simulink model "PhysicalEverSimmer"  (R2026a)
settings: Solver=VariableStepAuto  StopTime=14400
undefined symbols (not defined in the file or in its folder): ES_PackRate_bph, ES_PrepRate_bph, ES_QCRate_bph, ES_Resupply_bph, Fault_T_Cell1, Fault_T_Cell2, Fault_T_Cell3, Recipe_Block_s, Recipe_Count, Resupply_Cutoff_T, Transport_Latency_s, Transport_Rate_bph
(part 1 of 2)
settings Model: DataDictionary=PhysicalEverSimmerData.sldd  Creator=sarah  LastModifiedBy=sarah

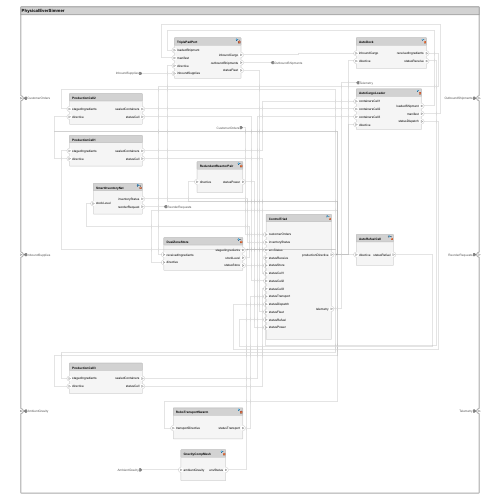
[thumbnail: Simulink's stored preview of the top-level diagram]
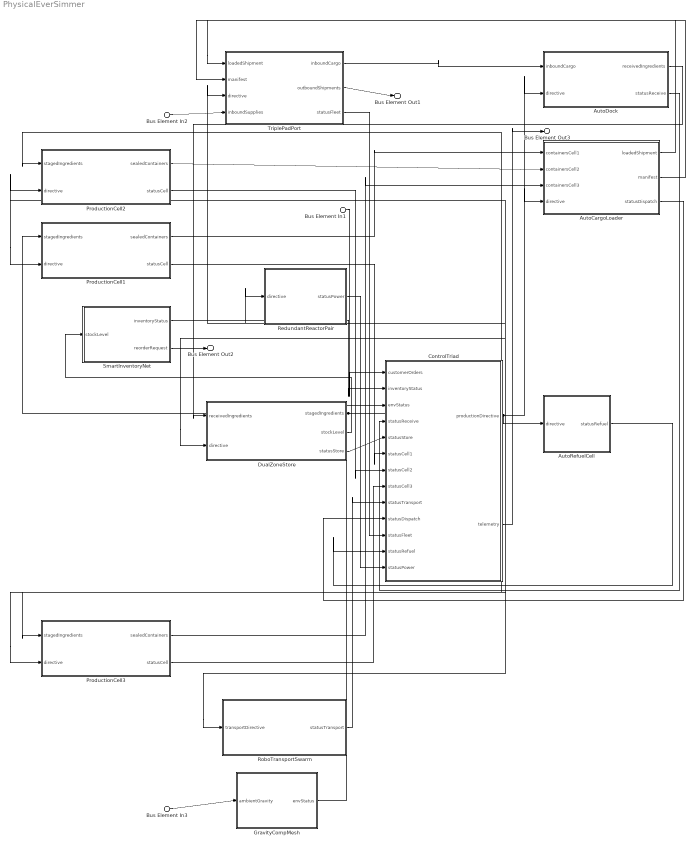
== system PhysicalEverSimmer ==
  Bus Element In1 : Inport  PortName=CustomerOrders
  Bus Element In2 : Inport  Port=2  PortName=InboundSupplies
  Bus Element In3 : Inport  Port=3  PortName=AmbientGravity
  AutoCargoLoader : Subsystem
      settings: PortSchema="{\"entries\":[{\"content\":{\"headerSize\":26,\"margin\":15,\"minimumSpacing\":25,\"sides\":[{\"content\":{\"connectorIds\":[\"In1\",\"In2\",\"In3\",\"In4\"]},\"type\":\"ConnectorPlacement.EquallySpacedRectSide\",\"uuid\":\"f830f98a-8e8b-4468-adf4-d6eab644987f\"},{\"content\":{\"connectorIds\":[\"Out1\",\"Out2\",\"Out3\"],\"side\":\"RIGHT\"},\"type\":\"ConnectorPlacement.EquallySpacedRectSide\",\"uuid\":\"7e0d0116-b3ba-4668-b638-30d0f54ba087\"},{\"content\":{\"side\":\"TOP\"},\"type\":\"ConnectorPlacement.EquallySpacedRectSide\",\"uuid\":\"7b4146d3-46d2-45ca-8c34-b106f0d8cedd\"}]},\"type\":\"ConnectorPlacement.EquallySpacedConnector\",\"uuid\":\"3d911b2d-a78f-42ea-b869-5e09982d9f54\"}],\"packageUris\":[\"http://schema.mathworks.com/mf0/Connector/R2020b\"],\"version\":\"1.0\"}"
  AutoDock : Subsystem
      settings: PortSchema="{\"entries\":[{\"content\":{\"headerSize\":26,\"margin\":15,\"minimumSpacing\":25,\"sides\":[{\"content\":{\"connectorIds\":[\"In1\",\"In2\"]},\"type\":\"ConnectorPlacement.EquallySpacedRectSide\",\"uuid\":\"f830f98a-8e8b-4468-adf4-d6eab644987f\"},{\"content\":{\"connectorIds\":[\"Out1\",\"Out2\"],\"side\":\"RIGHT\"},\"type\":\"ConnectorPlacement.EquallySpacedRectSide\",\"uuid\":\"7e0d0116-b3ba-4668-b638-30d0f54ba087\"},{\"content\":{\"side\":\"TOP\"},\"type\":\"ConnectorPlacement.EquallySpacedRectSide\",\"uuid\":\"7b4146d3-46d2-45ca-8c34-b106f0d8cedd\"}]},\"type\":\"ConnectorPlacement.EquallySpacedConnector\",\"uuid\":\"3d911b2d-a78f-42ea-b869-5e09982d9f54\"}],\"packageUris\":[\"http://schema.mathworks.com/mf0/Connector/R2020b\"],\"version\":\"1.0\"}"
  AutoRefuelCell : Subsystem
      settings: PortSchema="{\"entries\":[{\"content\":{\"headerSize\":26,\"margin\":15,\"minimumSpacing\":25,\"sides\":[{\"content\":{\"connectorIds\":[\"In1\"]},\"type\":\"ConnectorPlacement.EquallySpacedRectSide\",\"uuid\":\"f830f98a-8e8b-4468-adf4-d6eab644987f\"},{\"content\":{\"connectorIds\":[\"Out1\"],\"side\":\"RIGHT\"},\"type\":\"ConnectorPlacement.EquallySpacedRectSide\",\"uuid\":\"7e0d0116-b3ba-4668-b638-30d0f54ba087\"},{\"content\":{\"side\":\"TOP\"},\"type\":\"ConnectorPlacement.EquallySpacedRectSide\",\"uuid\":\"7b4146d3-46d2-45ca-8c34-b106f0d8cedd\"}]},\"type\":\"ConnectorPlacement.EquallySpacedConnector\",\"uuid\":\"3d911b2d-a78f-42ea-b869-5e09982d9f54\"}],\"packageUris\":[\"http://schema.mathworks.com/mf0/Connector/R2020b\"],\"version\":\"1.0\"}"
  ControlTriad : Subsystem
      settings: PortSchema="{\"entries\":[{\"content\":{\"headerSize\":26,\"margin\":15,\"minimumSpacing\":25,\"sides\":[{\"content\":{\"connectorIds\":[\"In1\",\"In2\",\"In3\",\"In4\",\"In5\",\"In6\",\"In7\",\"In8\",\"In9\",\"In10\",\"In11\",\"In12\",\"In13\"]},\"type\":\"ConnectorPlacement.EquallySpacedRectSide\",\"uuid\":\"f830f98a-8e8b-4468-adf4-d6eab644987f\"},{\"content\":{\"connectorIds\":[\"Out1\",\"Out2\"],\"side\":\"RIGHT\"},\"type\":\"ConnectorPlacement.EquallySpacedRectSide\",\"uuid\":\"7e0d0116-b3ba-4668-b638-30d0f54ba087\"},{\"content\":{\"side\":\"TOP\"},\"type\":\"ConnectorPlacement.EquallySpacedRectSide\",\"uuid\":\"7b4146d3-46d2-45ca-8c34-b106f0d8cedd\"}]},\"type\":\"ConnectorPlacement.EquallySpacedConnector\",\"uuid\":\"3d911b2d-a78f-42ea-b869-5e09982d9f54\"}],\"packageUris\":[\"http://schema.mathworks.com/mf0/Connector/R2020b\"],\"version\":\"1.0\"}"
  DualZoneStore : Subsystem
      settings: PortSchema="{\"entries\":[{\"content\":{\"headerSize\":26,\"margin\":15,\"minimumSpacing\":25,\"sides\":[{\"content\":{\"connectorIds\":[\"In1\",\"In2\"]},\"type\":\"ConnectorPlacement.EquallySpacedRectSide\",\"uuid\":\"f830f98a-8e8b-4468-adf4-d6eab644987f\"},{\"content\":{\"connectorIds\":[\"Out1\",\"Out2\",\"Out3\"],\"side\":\"RIGHT\"},\"type\":\"ConnectorPlacement.EquallySpacedRectSide\",\"uuid\":\"7e0d0116-b3ba-4668-b638-30d0f54ba087\"},{\"content\":{\"side\":\"TOP\"},\"type\":\"ConnectorPlacement.EquallySpacedRectSide\",\"uuid\":\"7b4146d3-46d2-45ca-8c34-b106f0d8cedd\"}]},\"type\":\"ConnectorPlacement.EquallySpacedConnector\",\"uuid\":\"3d911b2d-a78f-42ea-b869-5e09982d9f54\"}],\"packageUris\":[\"http://schema.mathworks.com/mf0/Connector/R2020b\"],\"version\":\"1.0\"}"
  GravityCompMesh : Subsystem
      settings: PortSchema="{\"entries\":[{\"content\":{\"headerSize\":26,\"margin\":15,\"minimumSpacing\":25,\"sides\":[{\"content\":{\"connectorIds\":[\"In1\"]},\"type\":\"ConnectorPlacement.EquallySpacedRectSide\",\"uuid\":\"f830f98a-8e8b-4468-adf4-d6eab644987f\"},{\"content\":{\"connectorIds\":[\"Out1\"],\"side\":\"RIGHT\"},\"type\":\"ConnectorPlacement.EquallySpacedRectSide\",\"uuid\":\"7e0d0116-b3ba-4668-b638-30d0f54ba087\"},{\"content\":{\"side\":\"TOP\"},\"type\":\"ConnectorPlacement.EquallySpacedRectSide\",\"uuid\":\"7b4146d3-46d2-45ca-8c34-b106f0d8cedd\"}]},\"type\":\"ConnectorPlacement.EquallySpacedConnector\",\"uuid\":\"3d911b2d-a78f-42ea-b869-5e09982d9f54\"}],\"packageUris\":[\"http://schema.mathworks.com/mf0/Connector/R2020b\"],\"version\":\"1.0\"}"
  ProductionCell1 : Subsystem
      settings: PortSchema="{\"entries\":[{\"content\":{\"headerSize\":26,\"margin\":15,\"minimumSpacing\":25,\"sides\":[{\"content\":{\"connectorIds\":[\"In1\",\"In2\"]},\"type\":\"ConnectorPlacement.EquallySpacedRectSide\",\"uuid\":\"f830f98a-8e8b-4468-adf4-d6eab644987f\"},{\"content\":{\"connectorIds\":[\"Out1\",\"Out2\"],\"side\":\"RIGHT\"},\"type\":\"ConnectorPlacement.EquallySpacedRectSide\",\"uuid\":\"7e0d0116-b3ba-4668-b638-30d0f54ba087\"},{\"content\":{\"side\":\"TOP\"},\"type\":\"ConnectorPlacement.EquallySpacedRectSide\",\"uuid\":\"7b4146d3-46d2-45ca-8c34-b106f0d8cedd\"}]},\"type\":\"ConnectorPlacement.EquallySpacedConnector\",\"uuid\":\"3d911b2d-a78f-42ea-b869-5e09982d9f54\"}],\"packageUris\":[\"http://schema.mathworks.com/mf0/Connector/R2020b\"],\"version\":\"1.0\"}"
  ProductionCell2 : Subsystem
      settings: PortSchema="{\"entries\":[{\"content\":{\"headerSize\":26,\"margin\":15,\"minimumSpacing\":25,\"sides\":[{\"content\":{\"connectorIds\":[\"In1\",\"In2\"]},\"type\":\"ConnectorPlacement.EquallySpacedRectSide\",\"uuid\":\"f830f98a-8e8b-4468-adf4-d6eab644987f\"},{\"content\":{\"connectorIds\":[\"Out1\",\"Out2\"],\"side\":\"RIGHT\"},\"type\":\"ConnectorPlacement.EquallySpacedRectSide\",\"uuid\":\"7e0d0116-b3ba-4668-b638-30d0f54ba087\"},{\"content\":{\"side\":\"TOP\"},\"type\":\"ConnectorPlacement.EquallySpacedRectSide\",\"uuid\":\"7b4146d3-46d2-45ca-8c34-b106f0d8cedd\"}]},\"type\":\"ConnectorPlacement.EquallySpacedConnector\",\"uuid\":\"3d911b2d-a78f-42ea-b869-5e09982d9f54\"}],\"packageUris\":[\"http://schema.mathworks.com/mf0/Connector/R2020b\"],\"version\":\"1.0\"}"
  ProductionCell3 : Subsystem
      settings: PortSchema="{\"entries\":[{\"content\":{\"headerSize\":26,\"margin\":15,\"minimumSpacing\":25,\"sides\":[{\"content\":{\"connectorIds\":[\"In1\",\"In2\"]},\"type\":\"ConnectorPlacement.EquallySpacedRectSide\",\"uuid\":\"f830f98a-8e8b-4468-adf4-d6eab644987f\"},{\"content\":{\"connectorIds\":[\"Out1\",\"Out2\"],\"side\":\"RIGHT\"},\"type\":\"ConnectorPlacement.EquallySpacedRectSide\",\"uuid\":\"7e0d0116-b3ba-4668-b638-30d0f54ba087\"},{\"content\":{\"side\":\"TOP\"},\"type\":\"ConnectorPlacement.EquallySpacedRectSide\",\"uuid\":\"7b4146d3-46d2-45ca-8c34-b106f0d8cedd\"}]},\"type\":\"ConnectorPlacement.EquallySpacedConnector\",\"uuid\":\"3d911b2d-a78f-42ea-b869-5e09982d9f54\"}],\"packageUris\":[\"http://schema.mathworks.com/mf0/Connector/R2020b\"],\"version\":\"1.0\"}"
  RedundantReactorPair : Subsystem
      settings: PortSchema="{\"entries\":[{\"content\":{\"headerSize\":26,\"margin\":15,\"minimumSpacing\":25,\"sides\":[{\"content\":{\"connectorIds\":[\"In1\"]},\"type\":\"ConnectorPlacement.EquallySpacedRectSide\",\"uuid\":\"f830f98a-8e8b-4468-adf4-d6eab644987f\"},{\"content\":{\"connectorIds\":[\"Out1\"],\"side\":\"RIGHT\"},\"type\":\"ConnectorPlacement.EquallySpacedRectSide\",\"uuid\":\"7e0d0116-b3ba-4668-b638-30d0f54ba087\"},{\"content\":{\"side\":\"TOP\"},\"type\":\"ConnectorPlacement.EquallySpacedRectSide\",\"uuid\":\"7b4146d3-46d2-45ca-8c34-b106f0d8cedd\"}]},\"type\":\"ConnectorPlacement.EquallySpacedConnector\",\"uuid\":\"3d911b2d-a78f-42ea-b869-5e09982d9f54\"}],\"packageUris\":[\"http://schema.mathworks.com/mf0/Connector/R2020b\"],\"version\":\"1.0\"}"
  RoboTransportSwarm : Subsystem
      settings: PortSchema="{\"entries\":[{\"content\":{\"headerSize\":26,\"margin\":15,\"minimumSpacing\":25,\"sides\":[{\"content\":{\"connectorIds\":[\"In1\"]},\"type\":\"ConnectorPlacement.EquallySpacedRectSide\",\"uuid\":\"f830f98a-8e8b-4468-adf4-d6eab644987f\"},{\"content\":{\"connectorIds\":[\"Out1\"],\"side\":\"RIGHT\"},\"type\":\"ConnectorPlacement.EquallySpacedRectSide\",\"uuid\":\"7e0d0116-b3ba-4668-b638-30d0f54ba087\"},{\"content\":{\"side\":\"TOP\"},\"type\":\"ConnectorPlacement.EquallySpacedRectSide\",\"uuid\":\"7b4146d3-46d2-45ca-8c34-b106f0d8cedd\"}]},\"type\":\"ConnectorPlacement.EquallySpacedConnector\",\"uuid\":\"3d911b2d-a78f-42ea-b869-5e09982d9f54\"}],\"packageUris\":[\"http://schema.mathworks.com/mf0/Connector/R2020b\"],\"version\":\"1.0\"}"
  SmartInventoryNet : Subsystem
      settings: PortSchema="{\"entries\":[{\"content\":{\"headerSize\":26,\"margin\":15,\"minimumSpacing\":25,\"sides\":[{\"content\":{\"connectorIds\":[\"In1\"]},\"type\":\"ConnectorPlacement.EquallySpacedRectSide\",\"uuid\":\"f830f98a-8e8b-4468-adf4-d6eab644987f\"},{\"content\":{\"connectorIds\":[\"Out1\",\"Out2\"],\"side\":\"RIGHT\"},\"type\":\"ConnectorPlacement.EquallySpacedRectSide\",\"uuid\":\"7e0d0116-b3ba-4668-b638-30d0f54ba087\"},{\"content\":{\"side\":\"TOP\"},\"type\":\"ConnectorPlacement.EquallySpacedRectSide\",\"uuid\":\"7b4146d3-46d2-45ca-8c34-b106f0d8cedd\"}]},\"type\":\"ConnectorPlacement.EquallySpacedConnector\",\"uuid\":\"3d911b2d-a78f-42ea-b869-5e09982d9f54\"}],\"packageUris\":[\"http://schema.mathworks.com/mf0/Connector/R2020b\"],\"version\":\"1.0\"}"
  TriplePadPort : Subsystem
      settings: PortSchema="{\"entries\":[{\"content\":{\"headerSize\":26,\"margin\":15,\"minimumSpacing\":25,\"sides\":[{\"content\":{\"connectorIds\":[\"In1\",\"In2\",\"In3\",\"In4\"]},\"type\":\"ConnectorPlacement.EquallySpacedRectSide\",\"uuid\":\"f830f98a-8e8b-4468-adf4-d6eab644987f\"},{\"content\":{\"connectorIds\":[\"Out1\",\"Out2\",\"Out3\"],\"side\":\"RIGHT\"},\"type\":\"ConnectorPlacement.EquallySpacedRectSide\",\"uuid\":\"7e0d0116-b3ba-4668-b638-30d0f54ba087\"},{\"content\":{\"side\":\"TOP\"},\"type\":\"ConnectorPlacement.EquallySpacedRectSide\",\"uuid\":\"7b4146d3-46d2-45ca-8c34-b106f0d8cedd\"}]},\"type\":\"ConnectorPlacement.EquallySpacedConnector\",\"uuid\":\"3d911b2d-a78f-42ea-b869-5e09982d9f54\"}],\"packageUris\":[\"http://schema.mathworks.com/mf0/Connector/R2020b\"],\"version\":\"1.0\"}"
  Bus Element Out1 : Outport  PortName=OutboundShipments
  Bus Element Out2 : Outport  Port=2  PortName=ReorderRequests
  Bus Element Out3 : Outport  Port=3  PortName=Telemetry
  wires:
  ProductionCell3/1(sealedContainers) -> AutoCargoLoader/3(containersCell3)
  ProductionCell1/2(statusCell) -> ControlTriad/6(statusCell1)
  Bus Element In2/1 -> TriplePadPort/4(inboundSupplies)
  DualZoneStore/2(stockLevel) -> SmartInventoryNet/1(stockLevel)
  SmartInventoryNet/1(inventoryStatus) -> ControlTriad/2(inventoryStatus)
  ProductionCell2/1(sealedContainers) -> AutoCargoLoader/2(containersCell2)
  ProductionCell2/2(statusCell) -> ControlTriad/7(statusCell2)
  SmartInventoryNet/2(reorderRequest) -> Bus Element Out2/1
  ProductionCell1/1(sealedContainers) -> AutoCargoLoader/1(containersCell1)
  ProductionCell3/2(statusCell) -> ControlTriad/8(statusCell3)
  Bus Element In3/1 -> GravityCompMesh/1(ambientGravity)
  RedundantReactorPair/1(statusPower) -> ControlTriad/13(statusPower)
  TriplePadPort/1(inboundCargo) -> AutoDock/1(inboundCargo)
  TriplePadPort/2(outboundShipments) -> Bus Element Out1/1
  TriplePadPort/3(statusFleet) -> ControlTriad/11(statusFleet)
  Bus Element In1/1 -> ControlTriad/1(customerOrders)
  AutoRefuelCell/1(statusRefuel) -> ControlTriad/12(statusRefuel)
  DualZoneStore/1(stagedIngredients) -> ProductionCell1/1(stagedIngredients), ProductionCell3/1(stagedIngredients), ProductionCell2/1(stagedIngredients)
  DualZoneStore/3(statusStore) -> ControlTriad/5(statusStore)
  AutoCargoLoader/1(loadedShipment) -> TriplePadPort/1(loadedShipment)
  RoboTransportSwarm/1(statusTransport) -> ControlTriad/9(statusTransport)
  GravityCompMesh/1(envStatus) -> ControlTriad/3(envStatus)
  ControlTriad/1(productionDirective) -> TriplePadPort/3(directive), ProductionCell1/2(directive), ProductionCell2/2(directive), RoboTransportSwarm/1(transportDirective), ProductionCell3/2(directive), DualZoneStore/2(directive), RedundantReactorPair/1(directive), AutoCargoLoader/4(directive), AutoDock/2(directive), AutoRefuelCell/1(directive)
  ControlTriad/2(telemetry) -> Bus Element Out3/1
  AutoDock/1(receivedIngredients) -> DualZoneStore/1(receivedIngredients)
  AutoDock/2(statusReceive) -> ControlTriad/4(statusReceive)
  AutoCargoLoader/2(manifest) -> TriplePadPort/2(manifest)
  AutoCargoLoader/3(statusDispatch) -> ControlTriad/10(statusDispatch)

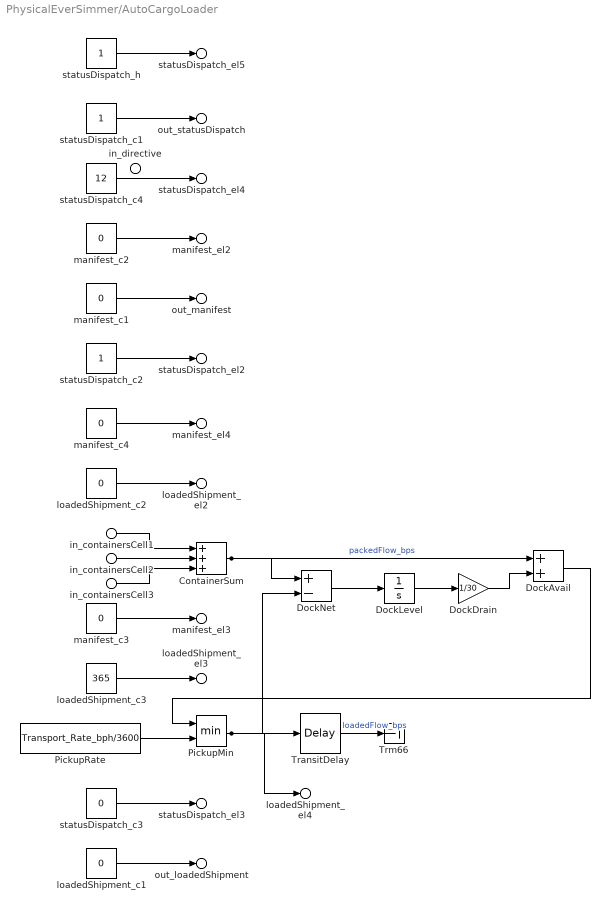
== system PhysicalEverSimmer/AutoCargoLoader ==
  in_containersCell1 : Inport  PortName=containersCell1  Element=flow_bps
  in_containersCell2 : Inport  Port=2  PortName=containersCell2  Element=flow_bps
  in_containersCell3 : Inport  Port=3  PortName=containersCell3  Element=flow_bps
  in_directive : Inport  Port=4  PortName=directive
  ContainerSum : Sum  Inputs=+++
  DockAvail : Sum
  DockDrain : Gain  Gain=1/30
  DockLevel : Integrator  LimitOutput=on  UpperSaturationLimit=600  LowerSaturationLimit=0
  DockNet : Sum  Inputs=+-
  PickupMin : MinMax  Inputs=2
  PickupRate : Constant  Value=Transport_Rate_bph/3600
  TransitDelay : TransportDelay  DelayTime=Transport_Latency_s
  Trm66 : Terminator
  loadedShipment_c1 : Constant  Value=0
  loadedShipment_c2 : Constant  Value=0
  loadedShipment_c3 : Constant  Value=365
  manifest_c{1..4} (4 alike) : Constant  Value=0
  statusDispatch_c1 : Constant
  statusDispatch_c2 : Constant
  statusDispatch_c3 : Constant  Value=0
  statusDispatch_c4 : Constant  Value=12
  statusDispatch_h : Constant
  out_loadedShipment : Outport  PortName=loadedShipment  Element=batchId
  loadedShipment_el2 : Outport  PortName=loadedShipment  Element=count
  loadedShipment_el3 : Outport  PortName=loadedShipment  Element=sealRating_days
  loadedShipment_el4 : Outport  PortName=loadedShipment  Element=flow_bps
  out_manifest : Outport  Port=2  PortName=manifest  Element=destinationId
  manifest_el2 : Outport  Port=2  PortName=manifest  Element=batchId
  manifest_el3 : Outport  Port=2  PortName=manifest  Element=count
  manifest_el4 : Outport  Port=2  PortName=manifest  Element=mass_kg
  out_statusDispatch : Outport  Port=3  PortName=statusDispatch  Element=unitId
  statusDispatch_el2 : Outport  Port=3  PortName=statusDispatch  Element=opState
  statusDispatch_el3 : Outport  Port=3  PortName=statusDispatch  Element=faultCode
  statusDispatch_el4 : Outport  Port=3  PortName=statusDispatch  Element=power_kW
  statusDispatch_el5 : Outport  Port=3  PortName=statusDispatch  Element=health
  wires:
  manifest_c4/1 -> manifest_el4/1
  ContainerSum/1 -> DockAvail/1, DockNet/1  "packedFlow_bps"
  statusDispatch_h/1 -> statusDispatch_el5/1
  loadedShipment_c2/1 -> loadedShipment_el2/1
  statusDispatch_c1/1 -> out_statusDispatch/1
  statusDispatch_c4/1 -> statusDispatch_el4/1
  statusDispatch_c2/1 -> statusDispatch_el2/1
  manifest_c2/1 -> manifest_el2/1
  manifest_c1/1 -> out_manifest/1
  in_containersCell1/1 -> ContainerSum/1
  in_containersCell2/1 -> ContainerSum/2
  in_containersCell3/1 -> ContainerSum/3
  manifest_c3/1 -> manifest_el3/1
  PickupMin/1 -> DockNet/2, loadedShipment_el4/1, TransitDelay/1
  loadedShipment_c3/1 -> loadedShipment_el3/1
  PickupRate/1 -> PickupMin/2
  statusDispatch_c3/1 -> statusDispatch_el3/1
  loadedShipment_c1/1 -> out_loadedShipment/1
  DockNet/1 -> DockLevel/1
  TransitDelay/1 -> Trm66/1  "loadedFlow_bps"
  DockLevel/1 -> DockDrain/1
  DockDrain/1 -> DockAvail/2
  DockAvail/1 -> PickupMin/1

== system PhysicalEverSimmer/AutoDock ==
  in_inboundCargo : Inport  PortName=inboundCargo  Element=flow_bps
  in_directive : Inport  Port=2  PortName=directive
  in_inboundCargoCap : Saturate  UpperLimit=0.0833333333333  LowerLimit=0
  receivedIngredients_c1 : Constant  Value=0
  receivedIngredients_c2 : Constant  Value=0
  receivedIngredients_c3 : Constant  Value=4
  statusReceive_c1 : Constant
  statusReceive_c2 : Constant
  statusReceive_c3 : Constant  Value=0
  statusReceive_c4 : Constant  Value=12
  statusReceive_h : Constant
  out_receivedIngredients : Outport  PortName=receivedIngredients  Element=palletId
  receivedIngredients_el2 : Outport  PortName=receivedIngredients  Element=mass_kg
  receivedIngredients_el3 : Outport  PortName=receivedIngredients  Element=temp_C
  receivedIngredients_el4 : Outport  PortName=receivedIngredients  Element=flow_bps
  out_statusReceive : Outport  Port=2  PortName=statusReceive  Element=unitId
  statusReceive_el2 : Outport  Port=2  PortName=statusReceive  Element=opState
  statusReceive_el3 : Outport  Port=2  PortName=statusReceive  Element=faultCode
  statusReceive_el4 : Outport  Port=2  PortName=statusReceive  Element=power_kW
  statusReceive_el5 : Outport  Port=2  PortName=statusReceive  Element=health
  wires:
  statusReceive_c4/1 -> statusReceive_el4/1
  receivedIngredients_c3/1 -> receivedIngredients_el3/1
  statusReceive_h/1 -> statusReceive_el5/1
  statusReceive_c1/1 -> out_statusReceive/1
  statusReceive_c2/1 -> statusReceive_el2/1
  in_inboundCargo/1 -> in_inboundCargoCap/1
  receivedIngredients_c2/1 -> receivedIngredients_el2/1
  receivedIngredients_c1/1 -> out_receivedIngredients/1
  statusReceive_c3/1 -> statusReceive_el3/1
  in_inboundCargoCap/1 -> receivedIngredients_el4/1

== system PhysicalEverSimmer/AutoRefuelCell ==
  in_directive : Inport  PortName=directive
  statusRefuel_c1 : Constant
  statusRefuel_c2 : Constant
  statusRefuel_c3 : Constant  Value=0
  statusRefuel_c4 : Constant  Value=10
  statusRefuel_h : Constant
  out_statusRefuel : Outport  PortName=statusRefuel  Element=unitId
  statusRefuel_el2 : Outport  PortName=statusRefuel  Element=opState
  statusRefuel_el3 : Outport  PortName=statusRefuel  Element=faultCode
  statusRefuel_el4 : Outport  PortName=statusRefuel  Element=power_kW
  statusRefuel_el5 : Outport  PortName=statusRefuel  Element=health
  wires:
  statusRefuel_c4/1 -> statusRefuel_el4/1
  statusRefuel_h/1 -> statusRefuel_el5/1
  statusRefuel_c1/1 -> out_statusRefuel/1
  statusRefuel_c3/1 -> statusRefuel_el3/1
  statusRefuel_c2/1 -> statusRefuel_el2/1

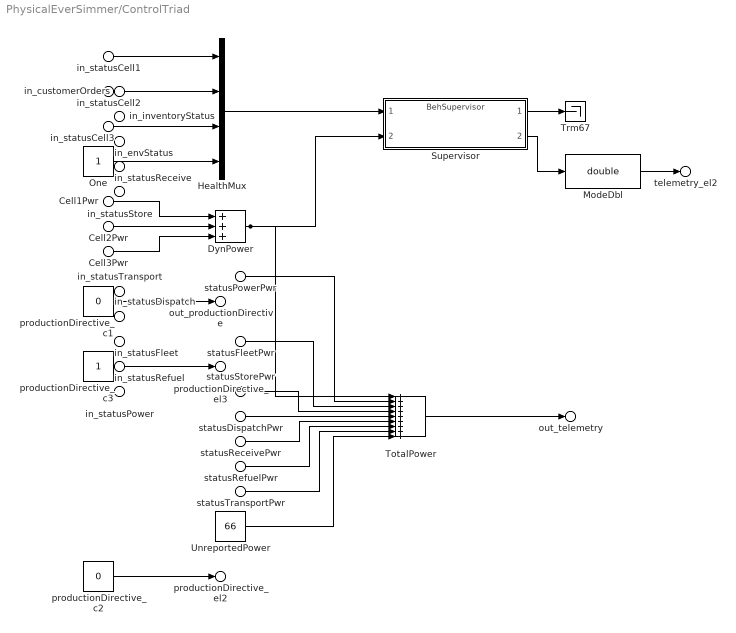
== system PhysicalEverSimmer/ControlTriad ==
  in_customerOrders : Inport  PortName=customerOrders
  in_inventoryStatus : Inport  Port=2  PortName=inventoryStatus
  in_envStatus : Inport  Port=3  PortName=envStatus
  in_statusReceive : Inport  Port=4  PortName=statusReceive
  statusReceivePwr : Inport  Port=4  PortName=statusReceive  Element=power_kW
  in_statusStore : Inport  Port=5  PortName=statusStore
  statusStorePwr : Inport  Port=5  PortName=statusStore  Element=power_kW
  Cell1Pwr : Inport  Port=6  PortName=statusCell1  Element=power_kW
  in_statusCell1 : Inport  Port=6  PortName=statusCell1  Element=health
  Cell2Pwr : Inport  Port=7  PortName=statusCell2  Element=power_kW
  in_statusCell2 : Inport  Port=7  PortName=statusCell2  Element=health
  Cell3Pwr : Inport  Port=8  PortName=statusCell3  Element=power_kW
  in_statusCell3 : Inport  Port=8  PortName=statusCell3  Element=health
  in_statusTransport : Inport  Port=9  PortName=statusTransport
  statusTransportPwr : Inport  Port=9  PortName=statusTransport  Element=power_kW
  in_statusDispatch : Inport  Port=10  PortName=statusDispatch
  statusDispatchPwr : Inport  Port=10  PortName=statusDispatch  Element=power_kW
  in_statusFleet : Inport  Port=11  PortName=statusFleet
  statusFleetPwr : Inport  Port=11  PortName=statusFleet  Element=power_kW
  in_statusRefuel : Inport  Port=12  PortName=statusRefuel
  statusRefuelPwr : Inport  Port=12  PortName=statusRefuel  Element=power_kW
  in_statusPower : Inport  Port=13  PortName=statusPower
  statusPowerPwr : Inport  Port=13  PortName=statusPower  Element=power_kW
  DynPower : Sum  Inputs=+++
  HealthMux : Mux
  ModeDbl : DataTypeConversion  OutDataTypeStr=double  SaturateOnIntegerOverflow=off  RndMeth=Floor
  One : Constant
  Supervisor : ModelReference  ModelNameDialog=BehSupervisor  ParameterArgumentNames=NumLines  ParameterArgumentValues=ES_NumLines  UsingDefaultArgumentValue=0  SimulationMode=Normal  ModelReferenceVersion=1.6
  TotalPower : Sum  Inputs=+++++++++
  Trm67 : Terminator
  UnreportedPower : Constant  Value=66
  productionDirective_c1 : Constant  Value=0
  productionDirective_c2 : Constant  Value=0
  productionDirective_c3 : Constant
  out_productionDirective : Outport  PortName=productionDirective  Element=cmdType
  productionDirective_el2 : Outport  PortName=productionDirective  Element=targetId
  productionDirective_el3 : Outport  PortName=productionDirective  Element=setpoint
  out_telemetry : Outport  Port=2  PortName=telemetry  Element=totalPower_kW
  telemetry_el2 : Outport  Port=2  PortName=telemetry  Element=plantMode
  wires:
  in_statusCell1/1 -> HealthMux/1
  Cell1Pwr/1 -> DynPower/1
  in_statusCell2/1 -> HealthMux/2
  in_statusCell3/1 -> HealthMux/3
  One/1 -> HealthMux/4
  Cell2Pwr/1 -> DynPower/2
  Cell3Pwr/1 -> DynPower/3
  productionDirective_c1/1 -> out_productionDirective/1
  productionDirective_c3/1 -> productionDirective_el3/1
  productionDirective_c2/1 -> productionDirective_el2/1
  HealthMux/1 -> Supervisor/1
  DynPower/1 -> Supervisor/2, TotalPower/1
  statusPowerPwr/1 -> TotalPower/2
  statusFleetPwr/1 -> TotalPower/3
  statusStorePwr/1 -> TotalPower/4
  statusDispatchPwr/1 -> TotalPower/5
  statusReceivePwr/1 -> TotalPower/6
  statusRefuelPwr/1 -> TotalPower/7
  statusTransportPwr/1 -> TotalPower/8
  UnreportedPower/1 -> TotalPower/9
  Supervisor/1 -> Trm67/1
  Supervisor/2 -> ModeDbl/1
  TotalPower/1 -> out_telemetry/1
  ModeDbl/1 -> telemetry_el2/1

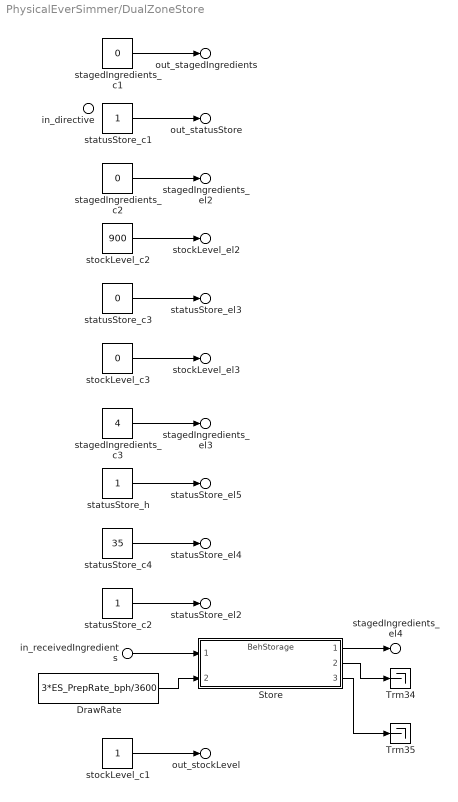
== system PhysicalEverSimmer/DualZoneStore ==
  in_receivedIngredients : Inport  PortName=receivedIngredients  Element=flow_bps
  in_directive : Inport  Port=2  PortName=directive  Element=setpoint
  DrawRate : Constant  Value=3*ES_PrepRate_bph/3600
  Store : ModelReference  ModelNameDialog=BehStorage  UsingDefaultArgumentValue=0,0  SimulationMode=Normal  ModelReferenceVersion=1.3
  Trm34 : Terminator
  Trm35 : Terminator
  stagedIngredients_c1 : Constant  Value=0
  stagedIngredients_c2 : Constant  Value=0
  stagedIngredients_c3 : Constant  Value=4
  statusStore_c1 : Constant
  statusStore_c2 : Constant
  statusStore_c3 : Constant  Value=0
  statusStore_c4 : Constant  Value=35
  statusStore_h : Constant
  stockLevel_c1 : Constant
  stockLevel_c2 : Constant  Value=900
  stockLevel_c3 : Constant  Value=0
  out_stagedIngredients : Outport  PortName=stagedIngredients  Element=palletId
  stagedIngredients_el2 : Outport  PortName=stagedIngredients  Element=mass_kg
  stagedIngredients_el3 : Outport  PortName=stagedIngredients  Element=temp_C
  stagedIngredients_el4 : Outport  PortName=stagedIngredients  Element=flow_bps
  out_stockLevel : Outport  Port=2  PortName=stockLevel  Element=itemId
  stockLevel_el2 : Outport  Port=2  PortName=stockLevel  Element=qty_units
  stockLevel_el3 : Outport  Port=2  PortName=stockLevel  Element=error_pct
  out_statusStore : Outport  Port=3  PortName=statusStore  Element=unitId
  statusStore_el2 : Outport  Port=3  PortName=statusStore  Element=opState
  statusStore_el3 : Outport  Port=3  PortName=statusStore  Element=faultCode
  statusStore_el4 : Outport  Port=3  PortName=statusStore  Element=power_kW
  statusStore_el5 : Outport  Port=3  PortName=statusStore  Element=health
  wires:
  stockLevel_c2/1 -> stockLevel_el2/1
  stagedIngredients_c3/1 -> stagedIngredients_el3/1
  stagedIngredients_c1/1 -> out_stagedIngredients/1
  in_receivedIngredients/1 -> Store/1
  stockLevel_c3/1 -> stockLevel_el3/1
  statusStore_c1/1 -> out_statusStore/1
  stagedIngredients_c2/1 -> stagedIngredients_el2/1
  statusStore_c3/1 -> statusStore_el3/1
  statusStore_h/1 -> statusStore_el5/1
  statusStore_c4/1 -> statusStore_el4/1
  statusStore_c2/1 -> statusStore_el2/1
  DrawRate/1 -> Store/2
  stockLevel_c1/1 -> out_stockLevel/1
  Store/1 -> stagedIngredients_el4/1
  Store/2 -> Trm34/1
  Store/3 -> Trm35/1

== system PhysicalEverSimmer/GravityCompMesh ==
  in_ambientGravity : Inport  PortName=ambientGravity  Element=gravity_g
  envStatus_c1 : Constant  Value=100
  out_envStatus : Outport  PortName=envStatus  Element=gravity_g
  envStatus_el2 : Outport  PortName=envStatus  Element=compensation_pct
  wires:
  in_ambientGravity/1 -> out_envStatus/1  "ambientGravity"
  envStatus_c1/1 -> envStatus_el2/1

== system PhysicalEverSimmer/ProductionCell1 ==
  Bus Element In1 : Inport  PortName=stagedIngredients
  Bus Element In2 : Inport  Port=2  PortName=directive
  CellController : Subsystem
      settings: PortSchema="{\"entries\":[{\"content\":{\"headerSize\":26,\"margin\":15,\"minimumSpacing\":25,\"sides\":[{\"content\":{\"connectorIds\":[\"In1\",\"In2\",\"In3\",\"In4\",\"In5\"]},\"type\":\"ConnectorPlacement.EquallySpacedRectSide\",\"uuid\":\"f830f98a-8e8b-4468-adf4-d6eab644987f\"},{\"content\":{\"connectorIds\":[\"Out1\",\"Out2\"],\"side\":\"RIGHT\"},\"type\":\"ConnectorPlacement.EquallySpacedRectSide\",\"uuid\":\"7e0d0116-b3ba-4668-b638-30d0f54ba087\"},{\"content\":{\"side\":\"TOP\"},\"type\":\"ConnectorPlacement.EquallySpacedRectSide\",\"uuid\":\"7b4146d3-46d2-45ca-8c34-b106f0d8cedd\"}]},\"type\":\"ConnectorPlacement.EquallySpacedConnector\",\"uuid\":\"3d911b2d-a78f-42ea-b869-5e09982d9f54\"}],\"packageUris\":[\"http://schema.mathworks.com/mf0/Connector/R2020b\"],\"version\":\"1.0\"}"
  CellCookVat : Subsystem
      settings: PortSchema="{\"entries\":[{\"content\":{\"headerSize\":26,\"margin\":15,\"minimumSpacing\":25,\"sides\":[{\"content\":{\"connectorIds\":[\"In1\",\"In2\"]},\"type\":\"ConnectorPlacement.EquallySpacedRectSide\",\"uuid\":\"f830f98a-8e8b-4468-adf4-d6eab644987f\"},{\"content\":{\"connectorIds\":[\"Out1\",\"Out2\"],\"side\":\"RIGHT\"},\"type\":\"ConnectorPlacement.EquallySpacedRectSide\",\"uuid\":\"7e0d0116-b3ba-4668-b638-30d0f54ba087\"},{\"content\":{\"side\":\"TOP\"},\"type\":\"ConnectorPlacement.EquallySpacedRectSide\",\"uuid\":\"7b4146d3-46d2-45ca-8c34-b106f0d8cedd\"}]},\"type\":\"ConnectorPlacement.EquallySpacedConnector\",\"uuid\":\"3d911b2d-a78f-42ea-b869-5e09982d9f54\"}],\"packageUris\":[\"http://schema.mathworks.com/mf0/Connector/R2020b\"],\"version\":\"1.0\"}"
  CellPackager : Subsystem
      settings: PortSchema="{\"entries\":[{\"content\":{\"headerSize\":26,\"margin\":15,\"minimumSpacing\":25,\"sides\":[{\"content\":{\"connectorIds\":[\"In1\",\"In2\"]},\"type\":\"ConnectorPlacement.EquallySpacedRectSide\",\"uuid\":\"f830f98a-8e8b-4468-adf4-d6eab644987f\"},{\"content\":{\"connectorIds\":[\"Out1\",\"Out2\"],\"side\":\"RIGHT\"},\"type\":\"ConnectorPlacement.EquallySpacedRectSide\",\"uuid\":\"7e0d0116-b3ba-4668-b638-30d0f54ba087\"},{\"content\":{\"side\":\"TOP\"},\"type\":\"ConnectorPlacement.EquallySpacedRectSide\",\"uuid\":\"7b4146d3-46d2-45ca-8c34-b106f0d8cedd\"}]},\"type\":\"ConnectorPlacement.EquallySpacedConnector\",\"uuid\":\"3d911b2d-a78f-42ea-b869-5e09982d9f54\"}],\"packageUris\":[\"http://schema.mathworks.com/mf0/Connector/R2020b\"],\"version\":\"1.0\"}"
  CellPrepUnit : Subsystem
      settings: PortSchema="{\"entries\":[{\"content\":{\"headerSize\":26,\"margin\":15,\"minimumSpacing\":25,\"sides\":[{\"content\":{\"connectorIds\":[\"In1\",\"In2\"]},\"type\":\"ConnectorPlacement.EquallySpacedRectSide\",\"uuid\":\"f830f98a-8e8b-4468-adf4-d6eab644987f\"},{\"content\":{\"connectorIds\":[\"Out1\",\"Out2\"],\"side\":\"RIGHT\"},\"type\":\"ConnectorPlacement.EquallySpacedRectSide\",\"uuid\":\"7e0d0116-b3ba-4668-b638-30d0f54ba087\"},{\"content\":{\"side\":\"TOP\"},\"type\":\"ConnectorPlacement.EquallySpacedRectSide\",\"uuid\":\"7b4146d3-46d2-45ca-8c34-b106f0d8cedd\"}]},\"type\":\"ConnectorPlacement.EquallySpacedConnector\",\"uuid\":\"3d911b2d-a78f-42ea-b869-5e09982d9f54\"}],\"packageUris\":[\"http://schema.mathworks.com/mf0/Connector/R2020b\"],\"version\":\"1.0\"}"
  CellQCSensor : Subsystem
      settings: PortSchema="{\"entries\":[{\"content\":{\"headerSize\":26,\"margin\":15,\"minimumSpacing\":25,\"sides\":[{\"content\":{\"connectorIds\":[\"In1\",\"In2\"]},\"type\":\"ConnectorPlacement.EquallySpacedRectSide\",\"uuid\":\"f830f98a-8e8b-4468-adf4-d6eab644987f\"},{\"content\":{\"connectorIds\":[\"Out1\",\"Out2\"],\"side\":\"RIGHT\"},\"type\":\"ConnectorPlacement.EquallySpacedRectSide\",\"uuid\":\"7e0d0116-b3ba-4668-b638-30d0f54ba087\"},{\"content\":{\"side\":\"TOP\"},\"type\":\"ConnectorPlacement.EquallySpacedRectSide\",\"uuid\":\"7b4146d3-46d2-45ca-8c34-b106f0d8cedd\"}]},\"type\":\"ConnectorPlacement.EquallySpacedConnector\",\"uuid\":\"3d911b2d-a78f-42ea-b869-5e09982d9f54\"}],\"packageUris\":[\"http://schema.mathworks.com/mf0/Connector/R2020b\"],\"version\":\"1.0\"}"
  Bus Element Out1 : Outport  PortName=sealedContainers
  Bus Element Out2 : Outport  Port=2  PortName=statusCell
  wires:
  Bus Element In1/1 -> CellPrepUnit/1(stagedIngredients)
  CellPrepUnit/1(preppedBatch) -> CellCookVat/1(preppedBatch)
  CellQCSensor/1(approvedSoup) -> CellPackager/1(approvedSoup)
  CellQCSensor/2(statusQA) -> CellController/4(statusQA)
  CellPrepUnit/2(statusPrep) -> CellController/2(statusPrep)
  CellPackager/1(sealedContainers) -> Bus Element Out1/1
  CellPackager/2(statusPack) -> CellController/5(statusPack)
  CellCookVat/1(cookedSoup) -> CellQCSensor/1(cookedSoup)
  CellCookVat/2(statusCook) -> CellController/3(statusCook)
  Bus Element In2/1 -> CellController/1(directive)
  CellController/1(cellDirective) -> CellQCSensor/2(directive), CellCookVat/2(directive), CellPackager/2(directive), CellPrepUnit/2(directive)
  CellController/2(statusCell) -> Bus Element Out2/1

== system PhysicalEverSimmer/ProductionCell2 ==
  Bus Element In1 : Inport  PortName=stagedIngredients
  Bus Element In2 : Inport  Port=2  PortName=directive
  CellController : Subsystem
      settings: PortSchema="{\"entries\":[{\"content\":{\"headerSize\":26,\"margin\":15,\"minimumSpacing\":25,\"sides\":[{\"content\":{\"connectorIds\":[\"In1\",\"In2\",\"In3\",\"In4\",\"In5\"]},\"type\":\"ConnectorPlacement.EquallySpacedRectSide\",\"uuid\":\"f830f98a-8e8b-4468-adf4-d6eab644987f\"},{\"content\":{\"connectorIds\":[\"Out1\",\"Out2\"],\"side\":\"RIGHT\"},\"type\":\"ConnectorPlacement.EquallySpacedRectSide\",\"uuid\":\"7e0d0116-b3ba-4668-b638-30d0f54ba087\"},{\"content\":{\"side\":\"TOP\"},\"type\":\"ConnectorPlacement.EquallySpacedRectSide\",\"uuid\":\"7b4146d3-46d2-45ca-8c34-b106f0d8cedd\"}]},\"type\":\"ConnectorPlacement.EquallySpacedConnector\",\"uuid\":\"3d911b2d-a78f-42ea-b869-5e09982d9f54\"}],\"packageUris\":[\"http://schema.mathworks.com/mf0/Connector/R2020b\"],\"version\":\"1.0\"}"
  CellCookVat : Subsystem
      settings: PortSchema="{\"entries\":[{\"content\":{\"headerSize\":26,\"margin\":15,\"minimumSpacing\":25,\"sides\":[{\"content\":{\"connectorIds\":[\"In1\",\"In2\"]},\"type\":\"ConnectorPlacement.EquallySpacedRectSide\",\"uuid\":\"f830f98a-8e8b-4468-adf4-d6eab644987f\"},{\"content\":{\"connectorIds\":[\"Out1\",\"Out2\"],\"side\":\"RIGHT\"},\"type\":\"ConnectorPlacement.EquallySpacedRectSide\",\"uuid\":\"7e0d0116-b3ba-4668-b638-30d0f54ba087\"},{\"content\":{\"side\":\"TOP\"},\"type\":\"ConnectorPlacement.EquallySpacedRectSide\",\"uuid\":\"7b4146d3-46d2-45ca-8c34-b106f0d8cedd\"}]},\"type\":\"ConnectorPlacement.EquallySpacedConnector\",\"uuid\":\"3d911b2d-a78f-42ea-b869-5e09982d9f54\"}],\"packageUris\":[\"http://schema.mathworks.com/mf0/Connector/R2020b\"],\"version\":\"1.0\"}"
  CellPackager : Subsystem
      settings: PortSchema="{\"entries\":[{\"content\":{\"headerSize\":26,\"margin\":15,\"minimumSpacing\":25,\"sides\":[{\"content\":{\"connectorIds\":[\"In1\",\"In2\"]},\"type\":\"ConnectorPlacement.EquallySpacedRectSide\",\"uuid\":\"f830f98a-8e8b-4468-adf4-d6eab644987f\"},{\"content\":{\"connectorIds\":[\"Out1\",\"Out2\"],\"side\":\"RIGHT\"},\"type\":\"ConnectorPlacement.EquallySpacedRectSide\",\"uuid\":\"7e0d0116-b3ba-4668-b638-30d0f54ba087\"},{\"content\":{\"side\":\"TOP\"},\"type\":\"ConnectorPlacement.EquallySpacedRectSide\",\"uuid\":\"7b4146d3-46d2-45ca-8c34-b106f0d8cedd\"}]},\"type\":\"ConnectorPlacement.EquallySpacedConnector\",\"uuid\":\"3d911b2d-a78f-42ea-b869-5e09982d9f54\"}],\"packageUris\":[\"http://schema.mathworks.com/mf0/Connector/R2020b\"],\"version\":\"1.0\"}"
  CellPrepUnit : Subsystem
      settings: PortSchema="{\"entries\":[{\"content\":{\"headerSize\":26,\"margin\":15,\"minimumSpacing\":25,\"sides\":[{\"content\":{\"connectorIds\":[\"In1\",\"In2\"]},\"type\":\"ConnectorPlacement.EquallySpacedRectSide\",\"uuid\":\"f830f98a-8e8b-4468-adf4-d6eab644987f\"},{\"content\":{\"connectorIds\":[\"Out1\",\"Out2\"],\"side\":\"RIGHT\"},\"type\":\"ConnectorPlacement.EquallySpacedRectSide\",\"uuid\":\"7e0d0116-b3ba-4668-b638-30d0f54ba087\"},{\"content\":{\"side\":\"TOP\"},\"type\":\"ConnectorPlacement.EquallySpacedRectSide\",\"uuid\":\"7b4146d3-46d2-45ca-8c34-b106f0d8cedd\"}]},\"type\":\"ConnectorPlacement.EquallySpacedConnector\",\"uuid\":\"3d911b2d-a78f-42ea-b869-5e09982d9f54\"}],\"packageUris\":[\"http://schema.mathworks.com/mf0/Connector/R2020b\"],\"version\":\"1.0\"}"
  CellQCSensor : Subsystem
      settings: PortSchema="{\"entries\":[{\"content\":{\"headerSize\":26,\"margin\":15,\"minimumSpacing\":25,\"sides\":[{\"content\":{\"connectorIds\":[\"In1\",\"In2\"]},\"type\":\"ConnectorPlacement.EquallySpacedRectSide\",\"uuid\":\"f830f98a-8e8b-4468-adf4-d6eab644987f\"},{\"content\":{\"connectorIds\":[\"Out1\",\"Out2\"],\"side\":\"RIGHT\"},\"type\":\"ConnectorPlacement.EquallySpacedRectSide\",\"uuid\":\"7e0d0116-b3ba-4668-b638-30d0f54ba087\"},{\"content\":{\"side\":\"TOP\"},\"type\":\"ConnectorPlacement.EquallySpacedRectSide\",\"uuid\":\"7b4146d3-46d2-45ca-8c34-b106f0d8cedd\"}]},\"type\":\"ConnectorPlacement.EquallySpacedConnector\",\"uuid\":\"3d911b2d-a78f-42ea-b869-5e09982d9f54\"}],\"packageUris\":[\"http://schema.mathworks.com/mf0/Connector/R2020b\"],\"version\":\"1.0\"}"
  Bus Element Out1 : Outport  PortName=sealedContainers
  Bus Element Out2 : Outport  Port=2  PortName=statusCell
  wires:
  CellPrepUnit/2(statusPrep) -> CellController/2(statusPrep)
  CellPrepUnit/1(preppedBatch) -> CellCookVat/1(preppedBatch)
  Bus Element In1/1 -> CellPrepUnit/1(stagedIngredients)
  CellQCSensor/1(approvedSoup) -> CellPackager/1(approvedSoup)
  CellQCSensor/2(statusQA) -> CellController/4(statusQA)
  Bus Element In2/1 -> CellController/1(directive)
  CellCookVat/1(cookedSoup) -> CellQCSensor/1(cookedSoup)
  CellCookVat/2(statusCook) -> CellController/3(statusCook)
  CellPackager/1(sealedContainers) -> Bus Element Out1/1
  CellPackager/2(statusPack) -> CellController/5(statusPack)
  CellController/1(cellDirective) -> CellCookVat/2(directive), CellQCSensor/2(directive), CellPrepUnit/2(directive), CellPackager/2(directive)
  CellController/2(statusCell) -> Bus Element Out2/1

== system PhysicalEverSimmer/ProductionCell3 ==
  Bus Element In1 : Inport  PortName=stagedIngredients
  Bus Element In2 : Inport  Port=2  PortName=directive
  CellController : Subsystem
      settings: PortSchema="{\"entries\":[{\"content\":{\"headerSize\":26,\"margin\":15,\"minimumSpacing\":25,\"sides\":[{\"content\":{\"connectorIds\":[\"In1\",\"In2\",\"In3\",\"In4\",\"In5\"]},\"type\":\"ConnectorPlacement.EquallySpacedRectSide\",\"uuid\":\"f830f98a-8e8b-4468-adf4-d6eab644987f\"},{\"content\":{\"connectorIds\":[\"Out1\",\"Out2\"],\"side\":\"RIGHT\"},\"type\":\"ConnectorPlacement.EquallySpacedRectSide\",\"uuid\":\"7e0d0116-b3ba-4668-b638-30d0f54ba087\"},{\"content\":{\"side\":\"TOP\"},\"type\":\"ConnectorPlacement.EquallySpacedRectSide\",\"uuid\":\"7b4146d3-46d2-45ca-8c34-b106f0d8cedd\"}]},\"type\":\"ConnectorPlacement.EquallySpacedConnector\",\"uuid\":\"3d911b2d-a78f-42ea-b869-5e09982d9f54\"}],\"packageUris\":[\"http://schema.mathworks.com/mf0/Connector/R2020b\"],\"version\":\"1.0\"}"
  CellCookVat : Subsystem
      settings: PortSchema="{\"entries\":[{\"content\":{\"headerSize\":26,\"margin\":15,\"minimumSpacing\":25,\"sides\":[{\"content\":{\"connectorIds\":[\"In1\",\"In2\"]},\"type\":\"ConnectorPlacement.EquallySpacedRectSide\",\"uuid\":\"f830f98a-8e8b-4468-adf4-d6eab644987f\"},{\"content\":{\"connectorIds\":[\"Out1\",\"Out2\"],\"side\":\"RIGHT\"},\"type\":\"ConnectorPlacement.EquallySpacedRectSide\",\"uuid\":\"7e0d0116-b3ba-4668-b638-30d0f54ba087\"},{\"content\":{\"side\":\"TOP\"},\"type\":\"ConnectorPlacement.EquallySpacedRectSide\",\"uuid\":\"7b4146d3-46d2-45ca-8c34-b106f0d8cedd\"}]},\"type\":\"ConnectorPlacement.EquallySpacedConnector\",\"uuid\":\"3d911b2d-a78f-42ea-b869-5e09982d9f54\"}],\"packageUris\":[\"http://schema.mathworks.com/mf0/Connector/R2020b\"],\"version\":\"1.0\"}"
  CellPackager : Subsystem
      settings: PortSchema="{\"entries\":[{\"content\":{\"headerSize\":26,\"margin\":15,\"minimumSpacing\":25,\"sides\":[{\"content\":{\"connectorIds\":[\"In1\",\"In2\"]},\"type\":\"ConnectorPlacement.EquallySpacedRectSide\",\"uuid\":\"f830f98a-8e8b-4468-adf4-d6eab644987f\"},{\"content\":{\"connectorIds\":[\"Out1\",\"Out2\"],\"side\":\"RIGHT\"},\"type\":\"ConnectorPlacement.EquallySpacedRectSide\",\"uuid\":\"7e0d0116-b3ba-4668-b638-30d0f54ba087\"},{\"content\":{\"side\":\"TOP\"},\"type\":\"ConnectorPlacement.EquallySpacedRectSide\",\"uuid\":\"7b4146d3-46d2-45ca-8c34-b106f0d8cedd\"}]},\"type\":\"ConnectorPlacement.EquallySpacedConnector\",\"uuid\":\"3d911b2d-a78f-42ea-b869-5e09982d9f54\"}],\"packageUris\":[\"http://schema.mathworks.com/mf0/Connector/R2020b\"],\"version\":\"1.0\"}"
  CellPrepUnit : Subsystem
      settings: PortSchema="{\"entries\":[{\"content\":{\"headerSize\":26,\"margin\":15,\"minimumSpacing\":25,\"sides\":[{\"content\":{\"connectorIds\":[\"In1\",\"In2\"]},\"type\":\"ConnectorPlacement.EquallySpacedRectSide\",\"uuid\":\"f830f98a-8e8b-4468-adf4-d6eab644987f\"},{\"content\":{\"connectorIds\":[\"Out1\",\"Out2\"],\"side\":\"RIGHT\"},\"type\":\"ConnectorPlacement.EquallySpacedRectSide\",\"uuid\":\"7e0d0116-b3ba-4668-b638-30d0f54ba087\"},{\"content\":{\"side\":\"TOP\"},\"type\":\"ConnectorPlacement.EquallySpacedRectSide\",\"uuid\":\"7b4146d3-46d2-45ca-8c34-b106f0d8cedd\"}]},\"type\":\"ConnectorPlacement.EquallySpacedConnector\",\"uuid\":\"3d911b2d-a78f-42ea-b869-5e09982d9f54\"}],\"packageUris\":[\"http://schema.mathworks.com/mf0/Connector/R2020b\"],\"version\":\"1.0\"}"
  CellQCSensor : Subsystem
      settings: PortSchema="{\"entries\":[{\"content\":{\"headerSize\":26,\"margin\":15,\"minimumSpacing\":25,\"sides\":[{\"content\":{\"connectorIds\":[\"In1\",\"In2\"]},\"type\":\"ConnectorPlacement.EquallySpacedRectSide\",\"uuid\":\"f830f98a-8e8b-4468-adf4-d6eab644987f\"},{\"content\":{\"connectorIds\":[\"Out1\",\"Out2\"],\"side\":\"RIGHT\"},\"type\":\"ConnectorPlacement.EquallySpacedRectSide\",\"uuid\":\"7e0d0116-b3ba-4668-b638-30d0f54ba087\"},{\"content\":{\"side\":\"TOP\"},\"type\":\"ConnectorPlacement.EquallySpacedRectSide\",\"uuid\":\"7b4146d3-46d2-45ca-8c34-b106f0d8cedd\"}]},\"type\":\"ConnectorPlacement.EquallySpacedConnector\",\"uuid\":\"3d911b2d-a78f-42ea-b869-5e09982d9f54\"}],\"packageUris\":[\"http://schema.mathworks.com/mf0/Connector/R2020b\"],\"version\":\"1.0\"}"
  Bus Element Out1 : Outport  PortName=sealedContainers
  Bus Element Out2 : Outport  Port=2  PortName=statusCell
  wires:
  Bus Element In1/1 -> CellPrepUnit/1(stagedIngredients)
  CellQCSensor/1(approvedSoup) -> CellPackager/1(approvedSoup)
  CellPrepUnit/1(preppedBatch) -> CellCookVat/1(preppedBatch)
  CellQCSensor/2(statusQA) -> CellController/4(statusQA)
  CellPrepUnit/2(statusPrep) -> CellController/2(statusPrep)
  CellCookVat/1(cookedSoup) -> CellQCSensor/1(cookedSoup)
  Bus Element In2/1 -> CellController/1(directive)
  CellCookVat/2(statusCook) -> CellController/3(statusCook)
  CellPackager/1(sealedContainers) -> Bus Element Out1/1
  CellPackager/2(statusPack) -> CellController/5(statusPack)
  CellController/1(cellDirective) -> CellCookVat/2(directive), CellPrepUnit/2(directive), CellPackager/2(directive), CellQCSensor/2(directive)
  CellController/2(statusCell) -> Bus Element Out2/1

== system PhysicalEverSimmer/RedundantReactorPair ==
  in_directive : Inport  PortName=directive
  statusPower_c1 : Constant
  statusPower_c2 : Constant
  statusPower_c3 : Constant  Value=0
  statusPower_c4 : Constant  Value=0
  statusPower_h : Constant
  out_statusPower : Outport  PortName=statusPower  Element=unitId
  statusPower_el2 : Outport  PortName=statusPower  Element=opState
  statusPower_el3 : Outport  PortName=statusPower  Element=faultCode
  statusPower_el4 : Outport  PortName=statusPower  Element=power_kW
  statusPower_el5 : Outport  PortName=statusPower  Element=health
  wires:
  statusPower_c1/1 -> out_statusPower/1
  statusPower_h/1 -> statusPower_el5/1
  statusPower_c3/1 -> statusPower_el3/1
  statusPower_c4/1 -> statusPower_el4/1
  statusPower_c2/1 -> statusPower_el2/1

== system PhysicalEverSimmer/RoboTransportSwarm ==
  in_transportDirective : Inport  PortName=transportDirective
  statusTransport_c1 : Constant
  statusTransport_c2 : Constant
  statusTransport_c3 : Constant  Value=0
  statusTransport_c4 : Constant  Value=15
  statusTransport_h : Constant
  out_statusTransport : Outport  PortName=statusTransport  Element=unitId
  statusTransport_el2 : Outport  PortName=statusTransport  Element=opState
  statusTransport_el3 : Outport  PortName=statusTransport  Element=faultCode
  statusTransport_el4 : Outport  PortName=statusTransport  Element=power_kW
  statusTransport_el5 : Outport  PortName=statusTransport  Element=health
  wires:
  statusTransport_c1/1 -> out_statusTransport/1
  statusTransport_h/1 -> statusTransport_el5/1
  statusTransport_c3/1 -> statusTransport_el3/1
  statusTransport_c4/1 -> statusTransport_el4/1
  statusTransport_c2/1 -> statusTransport_el2/1

== system PhysicalEverSimmer/SmartInventoryNet ==
  in_stockLevel : Inport  PortName=stockLevel
  inventoryStatus_c1 : Constant
  inventoryStatus_c2 : Constant  Value=900
  inventoryStatus_c3 : Constant  Value=0
  reorderRequest_c1 : Constant
  reorderRequest_c2 : Constant  Value=0
  reorderRequest_c3 : Constant  Value=0
  out_inventoryStatus : Outport  PortName=inventoryStatus  Element=itemId
  inventoryStatus_el2 : Outport  PortName=inventoryStatus  Element=qty_units
  inventoryStatus_el3 : Outport  PortName=inventoryStatus  Element=error_pct
  out_reorderRequest : Outport  Port=2  PortName=reorderRequest  Element=itemId
  reorderRequest_el2 : Outport  Port=2  PortName=reorderRequest  Element=qty_units
  reorderRequest_el3 : Outport  Port=2  PortName=reorderRequest  Element=error_pct
  wires:
  inventoryStatus_c1/1 -> out_inventoryStatus/1
  reorderRequest_c2/1 -> reorderRequest_el2/1
  inventoryStatus_c2/1 -> inventoryStatus_el2/1
  reorderRequest_c3/1 -> reorderRequest_el3/1
  inventoryStatus_c3/1 -> inventoryStatus_el3/1
  reorderRequest_c1/1 -> out_reorderRequest/1

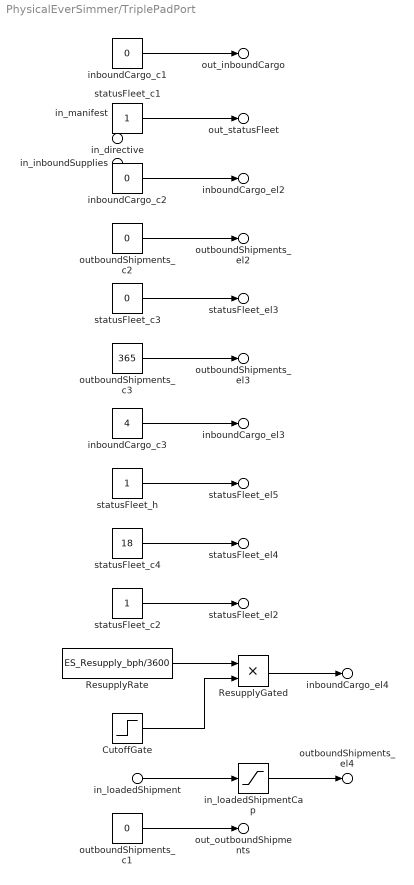
== system PhysicalEverSimmer/TriplePadPort ==
  in_loadedShipment : Inport  PortName=loadedShipment  Element=flow_bps
  in_manifest : Inport  Port=2  PortName=manifest
  in_directive : Inport  Port=3  PortName=directive
  in_inboundSupplies : Inport  Port=4  PortName=inboundSupplies
  CutoffGate : Step  Time=Resupply_Cutoff_T  InitialValue=1  FinalValue=0  SampleTime=0
  ResupplyGated : Product
  ResupplyRate : Constant  Value=ES_Resupply_bph/3600
  in_loadedShipmentCap : Saturate  UpperLimit=0.0777777777778  LowerLimit=0
  inboundCargo_c1 : Constant  Value=0
  inboundCargo_c2 : Constant  Value=0
  inboundCargo_c3 : Constant  Value=4
  outboundShipments_c1 : Constant  Value=0
  outboundShipments_c2 : Constant  Value=0
  outboundShipments_c3 : Constant  Value=365
  statusFleet_c1 : Constant
  statusFleet_c2 : Constant
  statusFleet_c3 : Constant  Value=0
  statusFleet_c4 : Constant  Value=18
  statusFleet_h : Constant
  out_inboundCargo : Outport  PortName=inboundCargo  Element=palletId
  inboundCargo_el2 : Outport  PortName=inboundCargo  Element=mass_kg
  inboundCargo_el3 : Outport  PortName=inboundCargo  Element=temp_C
  inboundCargo_el4 : Outport  PortName=inboundCargo  Element=flow_bps
  out_outboundShipments : Outport  Port=2  PortName=outboundShipments  Element=batchId
  outboundShipments_el2 : Outport  Port=2  PortName=outboundShipments  Element=count
  outboundShipments_el3 : Outport  Port=2  PortName=outboundShipments  Element=sealRating_days
  outboundShipments_el4 : Outport  Port=2  PortName=outboundShipments  Element=flow_bps
  out_statusFleet : Outport  Port=3  PortName=statusFleet  Element=unitId
  statusFleet_el2 : Outport  Port=3  PortName=statusFleet  Element=opState
  statusFleet_el3 : Outport  Port=3  PortName=statusFleet  Element=faultCode
  statusFleet_el4 : Outport  Port=3  PortName=statusFleet  Element=power_kW
  statusFleet_el5 : Outport  Port=3  PortName=statusFleet  Element=health
  wires:
  statusFleet_c3/1 -> statusFleet_el3/1
  outboundShipments_c2/1 -> outboundShipments_el2/1
  inboundCargo_c1/1 -> out_inboundCargo/1
  statusFleet_h/1 -> statusFleet_el5/1
  inboundCargo_c3/1 -> inboundCargo_el3/1
  statusFleet_c1/1 -> out_statusFleet/1
  outboundShipments_c3/1 -> outboundShipments_el3/1
  inboundCargo_c2/1 -> inboundCargo_el2/1
  statusFleet_c4/1 -> statusFleet_el4/1
  statusFleet_c2/1 -> statusFleet_el2/1
  ResupplyRate/1 -> ResupplyGated/1
  CutoffGate/1 -> ResupplyGated/2
  in_loadedShipment/1 -> in_loadedShipmentCap/1
  outboundShipments_c1/1 -> out_outboundShipments/1
  ResupplyGated/1 -> inboundCargo_el4/1
  in_loadedShipmentCap/1 -> outboundShipments_el4/1

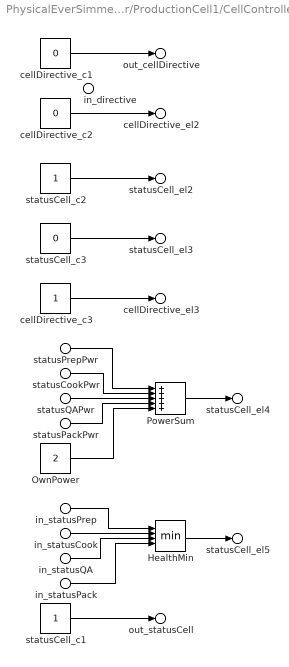
== system PhysicalEverSimmer/ProductionCell1/CellController ==
  in_directive : Inport  PortName=directive
  statusPrepPwr : Inport  Port=2  PortName=statusPrep  Element=power_kW
  in_statusPrep : Inport  Port=2  PortName=statusPrep  Element=health
  statusCookPwr : Inport  Port=3  PortName=statusCook  Element=power_kW
  in_statusCook : Inport  Port=3  PortName=statusCook  Element=health
  statusQAPwr : Inport  Port=4  PortName=statusQA  Element=power_kW
  in_statusQA : Inport  Port=4  PortName=statusQA  Element=health
  statusPackPwr : Inport  Port=5  PortName=statusPack  Element=power_kW
  in_statusPack : Inport  Port=5  PortName=statusPack  Element=health
  HealthMin : MinMax  Inputs=4
  OwnPower : Constant  Value=2
  PowerSum : Sum  Inputs=+++++
  cellDirective_c1 : Constant  Value=0
  cellDirective_c2 : Constant  Value=0
  cellDirective_c3 : Constant
  statusCell_c1 : Constant
  statusCell_c2 : Constant
  statusCell_c3 : Constant  Value=0
  out_cellDirective : Outport  PortName=cellDirective  Element=cmdType
  cellDirective_el2 : Outport  PortName=cellDirective  Element=targetId
  cellDirective_el3 : Outport  PortName=cellDirective  Element=setpoint
  out_statusCell : Outport  Port=2  PortName=statusCell  Element=unitId
  statusCell_el2 : Outport  Port=2  PortName=statusCell  Element=opState
  statusCell_el3 : Outport  Port=2  PortName=statusCell  Element=faultCode
  statusCell_el4 : Outport  Port=2  PortName=statusCell  Element=power_kW
  statusCell_el5 : Outport  Port=2  PortName=statusCell  Element=health
  wires:
  cellDirective_c1/1 -> out_cellDirective/1
  statusCookPwr/1 -> PowerSum/2
  cellDirective_c2/1 -> cellDirective_el2/1
  statusCell_c2/1 -> statusCell_el2/1
  statusCell_c3/1 -> statusCell_el3/1
  cellDirective_c3/1 -> cellDirective_el3/1
  statusPrepPwr/1 -> PowerSum/1
  statusQAPwr/1 -> PowerSum/3
  statusPackPwr/1 -> PowerSum/4
  OwnPower/1 -> PowerSum/5
  in_statusPrep/1 -> HealthMin/1
  in_statusCook/1 -> HealthMin/2
  in_statusQA/1 -> HealthMin/3
  in_statusPack/1 -> HealthMin/4
  statusCell_c1/1 -> out_statusCell/1
  PowerSum/1 -> statusCell_el4/1
  HealthMin/1 -> statusCell_el5/1
